simulink model "Linear_MPC_design"  (R2024a)
settings: Solver=VariableStepAuto  StartTime=0.0  StopTime=8  MaxStep=0.1  RelTol=1e-3
model workspace (MAT data in the model file):
  Sig = Simulink.Signal
  Sig.DataType = 'auto'
  Sig.Dimensions = -1
  Sig.DimensionsMode = 'auto'
  Sig.Complexity = 'auto'
  Sig.SampleTime = -1
  Sig.SamplingMode = 'auto'
undefined symbols (not defined in the file): Ts
libraries: Bonus_Library x3, cstblocks x1, mpcadaslib x1, mpclib x1
settings Model: PauseTimes=4  Creator=mulusoy  LastModifiedBy=User
settings OptimizationCC: ReuseModelBlockBuffer=off
settings RTWCC: GPUComputeCapability=3.5

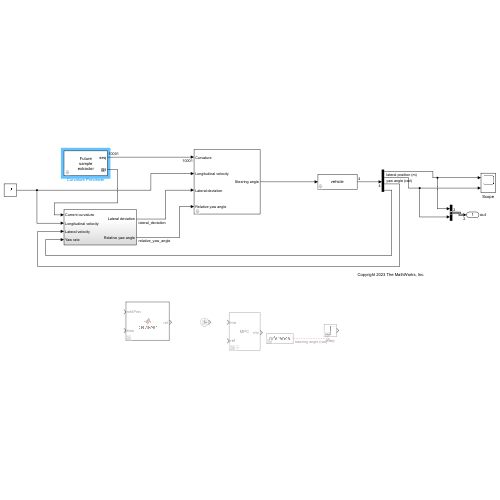
[thumbnail: Simulink's stored preview of the top-level diagram]
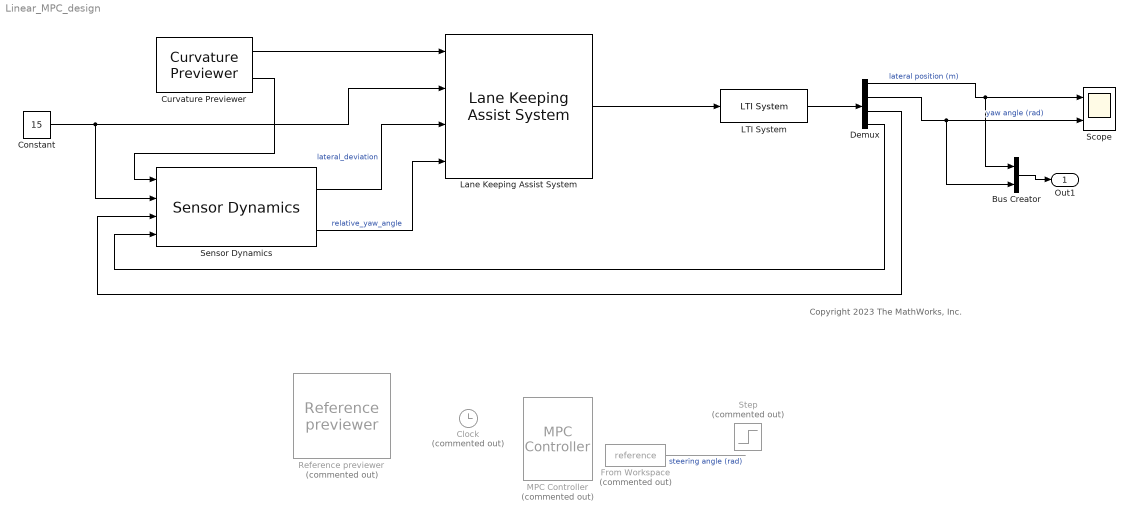
== system Linear_MPC_design ==
  note: Copyright 2023 The MathWorks, Inc.
  Bus Creator : BusCreator  Inputs=2
  Clock : Clock  Commented=on
  Constant : Constant  Value=15
  Curvature Previewer : Bonus_Library/Curvature Previewer  signal=md  ts=.001  steps=10000
  Demux : Demux
  From Workspace : FromWorkspace  Commented=on  VariableName=reference
  LTI System : cstblocks/LTI System  sys=vehicle  IC=[]  PadeOrder=0
  Lane Keeping Assist System : mpcadaslib/Lane Keeping Assist System  ModelType=Use vehicle parameters  VehicleMass=1575  VehicleYawInertia=2875  LengthToFront=1.2  LengthToRear=1.6  FrontTireStiffness=19000  RearTireStiffness=33000  EgoModelMatrixA=[-4.4021 ,-12.4603;1.3913,-5.1868]  EgoModelMatrixB=[24.1270;15.8609]  EgoModelMatrixC=[1,0;0,1]  InitialLongVel=15  TransportLag=0  MinSteering=-0.26  umin_ext=off  MaxSteering=0.26  umax_ext=off  Ts=.05  PredictionHorizon=14  ControllerBehavior=0.490  suboptimal=off  maxiter=10  datatypeopt=double  optmode=off  trackmode=off
      settings: LibrarySourceBlock=mpclib/Automated Driving/Lane Keeping Assist System
  MPC Controller : mpclib/MPC Controller  Commented=on  SCDEnableBlockLinearizationSpecification=on  is_multiple=0  enable_value=0  return_u0=off  updateMPCinCallerWorkspace=on  md_inport=off  mv_inport=off  uref_inport=off  return_cost=off  return_mvseq=off  return_qpstatus=off  return_xseq=off  return_state=off  return_ovseq=off  state_inport=off  umin_inport=off  umax_inport=off  ymin_inport=off  ymax_inport=off  cc_inport=off  ywt_inport=off  uwt_inport=off  duwt_inport=off  rhoeps_inport=off  pm_inport=off  MaximumP=10  HorizonChoice=FixedHorizon  n_ts=1  n_p=10  n_mv=1  n_md=1  n_ud=0  n_mo=2  n_uo=0  BlockDataType=double  SampleTimeInherited=off  switch_inport=off
  Reference previewer : Bonus_Library/Reference previewer  Commented=on  SystemSampleTime=Ts  VariantActivationTime=update diagram  AllowFlexibleInterface=on  Latency=0  AutoFrameSizeCalculation=off
  Scope : Scope  NumInputPorts=2
  Sensor Dynamics : Bonus_Library/Sensor Dynamics  SystemSampleTime=-1  VariantActivationTime=update diagram  AllowFlexibleInterface=on  Latency=0  AutoFrameSizeCalculation=off
  Step : Step  Commented=on  Time=4  After=pi/6  SampleTime=0
  Out1 : Outport  SignalName=out
  wires:
  LTI System/1 -> Demux/1
  From Workspace/1 -> ?  "steering angle (rad)"
  Curvature Previewer/1 -> Lane Keeping Assist System/1
  Constant/1 -> Sensor Dynamics/2, Lane Keeping Assist System/2
  Sensor Dynamics/1 -> Lane Keeping Assist System/3  "lateral_deviation"
  Sensor Dynamics/2 -> Lane Keeping Assist System/4  "relative_yaw_angle"
  Curvature Previewer/2 -> Sensor Dynamics/1
  Lane Keeping Assist System/1 -> LTI System/1
  Demux/1 -> Bus Creator/1, Scope/1  "lateral position (m)"
  Demux/2 -> Bus Creator/2, Scope/2  "yaw angle (rad)"
  Demux/3 -> Sensor Dynamics/3
  Demux/4 -> Sensor Dynamics/4
  Bus Creator/1 -> Out1/1
